simulink model "kalman_point_mass_1d"  (R2017a)
settings: Solver=FixedStepAuto  StartTime=0.0  StopTime=10  FixedStep=0.1  RelTol=1e-3
libraries: simulink x3
settings Model: Creator=jdam  LastModifiedBy=jdam

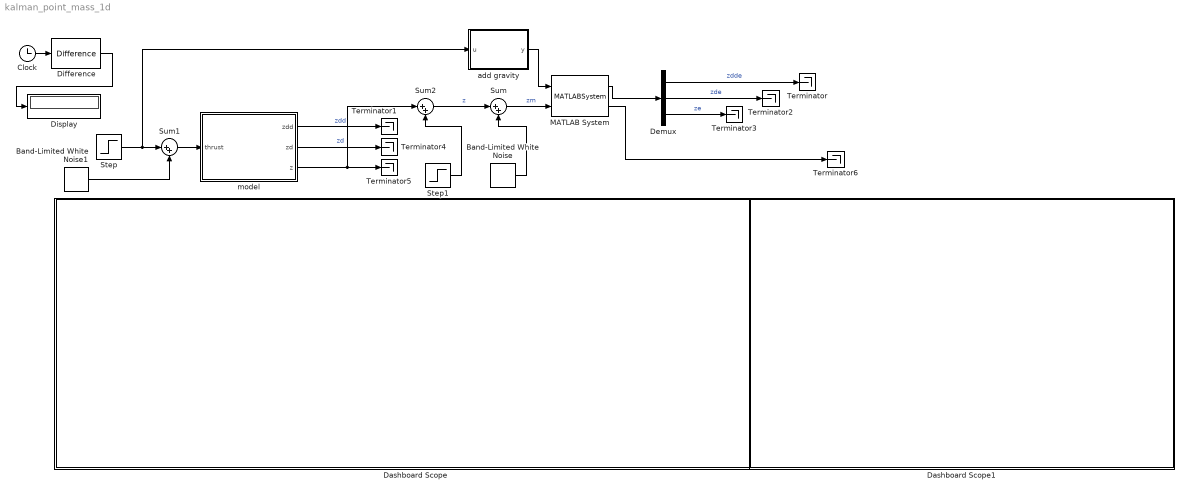
== system kalman_point_mass_1d ==
  Band-Limited White Noise : simulink/Sources/Band-Limited White Noise  Cov=[300]  Ts=0.1  seed=[23341]
  Band-Limited White Noise1 : simulink/Sources/Band-Limited White Noise  Cov=[10]  Ts=0.1  seed=[23341]
  Clock : Clock
  Dashboard Scope : Subsystem  DialogController=hmiCreateDDGDialog  IsWebBlock=on  mask(MWDashboardBlock){webBlockId=0870576e-867d-4307-93df-fca29635653f, webBlockType=sdiscope, ShowInitialText=on, HMISrcModelName=kalman_point_mass_1d}
      mask prompts: webBlockId "WebBlock Id"; webBlockType "WebBlock Type"; HMISrcModelName "Source Model"
      mask help: SimulinkHMI:dialogs:HMIScopeDialogDesc
      mask Help: helpview([docroot '/mapfiles/simulink.map'], 'hmi_scope')
      mask Display:
      | if strcmp(get_param(bdroot(gcb),'BlockDiagramType'), 'library')
      |     image([(matlabroot) '/toolbox/simulink/hmi/icons/DashboardScope.png']);
      | end
  Dashboard Scope1 : Subsystem  DialogController=hmiCreateDDGDialog  IsWebBlock=on  mask(MWDashboardBlock){webBlockId=ac143f71-d047-4cf6-8aa9-aa511e5f50dd, webBlockType=sdiscope, ShowInitialText=on, HMISrcModelName=kalman_point_mass_1d}
      mask prompts: webBlockId "WebBlock Id"; webBlockType "WebBlock Type"; HMISrcModelName "Source Model"
      mask help: SimulinkHMI:dialogs:HMIScopeDialogDesc
      mask Help: helpview([docroot '/mapfiles/simulink.map'], 'hmi_scope')
      mask Display:
      | if strcmp(get_param(bdroot(gcb),'BlockDiagramType'), 'library')
      |     image([(matlabroot) '/toolbox/simulink/hmi/icons/DashboardScope.png']);
      | end
  Demux : Demux  Outputs=3
  Difference : simulink/Discrete/Difference  ICPrevInput=0.0  OutMin=[]  OutMax=[]  OutDataType=fixdt(1, 16)  OutScaling=2^-10  DoSatur=off
  Display : Display
  MATLAB System : MATLABSystem  System=kalman  SimulateUsing=Interpreted execution
      mask Type: kalman
      mask Display:
      | disp('kalman');
      | port_label('input',1,'u');
      | port_label('input',2,'z');
      | port_label('output',1,'xe');
      | port_label('output',2,'P');
  Step : Step  Time=3  After=25  SampleTime=0
  Step1 : Step  Time=6  After=110.0  SampleTime=0
  Sum : Sum  Inputs=|++
  Sum1 : Sum  Inputs=|++
  Sum2 : Sum  Inputs=|++
  Terminator{,1..6} (7 alike) : Terminator
  add gravity : MATLAB Function  TreatAsAtomicUnit=on
  model : Subsystem
  wires:
  Step/1 -> Sum1/1, add gravity/1(u)
  Demux/1 -> Terminator/1  "zdde"
  Demux/2 -> Terminator2/1  "zde"
  Demux/3 -> Terminator3/1  "ze"
  MATLAB System/1 -> Demux/1
  add gravity/1(y) -> MATLAB System/1
  model/1(zdd) -> Terminator1/1  "zdd"
  model/2(zd) -> Terminator4/1  "zd"
  model/3(z) -> Sum2/1, Terminator5/1
  Difference/1 -> Display/1
  Clock/1 -> Difference/1
  Sum/1 -> MATLAB System/2  "zm"
  Sum1/1 -> model/1(thrust)
  Band-Limited White Noise1/1 -> Sum1/2
  Band-Limited White Noise/1 -> Sum/2
  Sum2/1 -> Sum/1  "z"
  Step1/1 -> Sum2/2
  MATLAB System/2 -> Terminator6/1

== system kalman_point_mass_1d/Dashboard Scope ==

== system kalman_point_mass_1d/Dashboard Scope1 ==

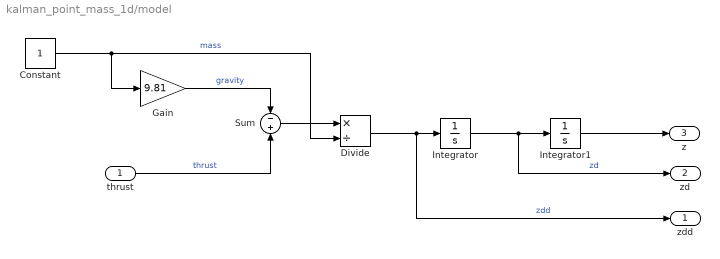
== system kalman_point_mass_1d/model ==
  thrust : Inport
  Constant : Constant
  Divide : Product  Inputs=*/
  Gain : Gain  Gain=9.81
  Integrator : Integrator
  Integrator1 : Integrator  InitialCondition=5
  Sum : Sum  Inputs=-|+
  zdd : Outport
  zd : Outport  Port=2
  z : Outport  Port=3
  wires:
  Sum/1 -> Divide/1
  Gain/1 -> Sum/1  "gravity"
  thrust/1 -> Sum/2  "thrust"
  Constant/1 -> Gain/1, Divide/2  "mass"
  Integrator/1 -> zd/1, Integrator1/1  "zd"
  Divide/1 -> zdd/1, Integrator/1  "zdd"
  Integrator1/1 -> z/1

== matlab function kalman_point_mass_1d/add gravity ==
  data: u input; y output
function y = fcn(u)
mass = 1;
F = u - mass*9.81;
y = F/mass;
